simulink model "gm_sampleModel2013_4_sub"  (R2023a)
settings: Solver=VariableStepAuto  StartTime=0.0  StopTime=10.0  RelTol=1e-3
libraries: simulink x1
settings Model: Creator=user1  LastModifiedBy=user1
settings OptimizationCC: BlockReduction=off  ConditionallyExecuteInputs=off
settings DebuggingCC: InheritedTsInSrcMsg=none

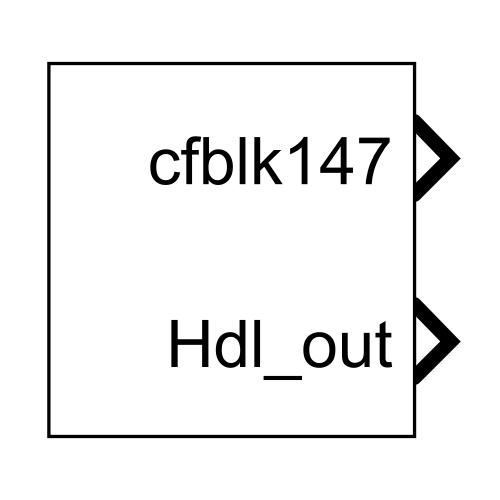
[thumbnail: Simulink's stored preview of the top-level diagram]
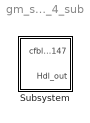
== system gm_sampleModel2013_4_sub ==
  Subsystem : Subsystem

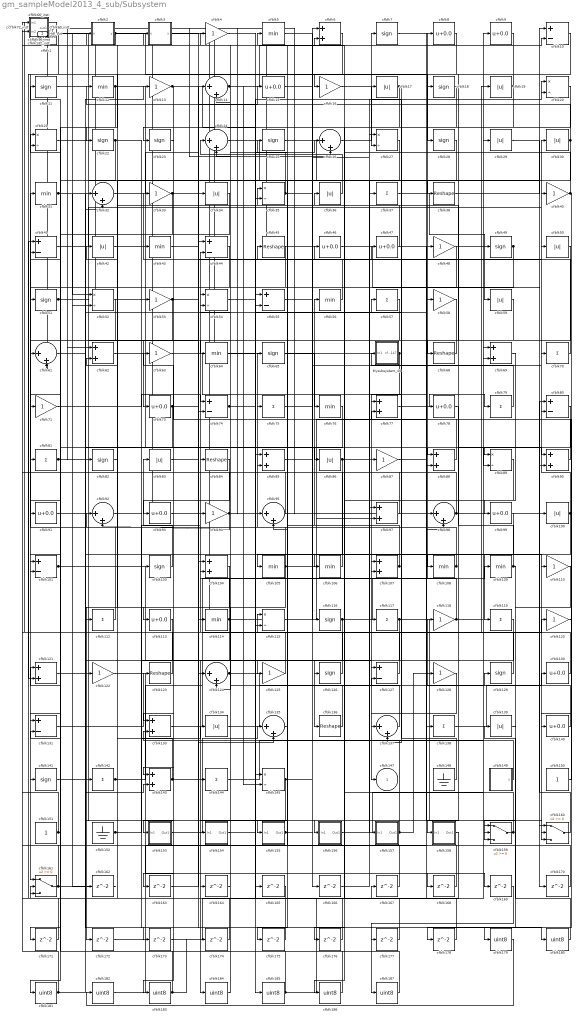
== system gm_sampleModel2013_4_sub/Subsystem ==
  Mysubsystem_45 : Subsystem
  cfblk1 : simulink/Logic and Bit Operations/Detect Increase  vinit=0.0  OutDataTypeStr=uint8
      settings: LibrarySourceBlock=|
      | hdlsllib/Logic and Bit
      | Operations/Detect
      | Increase
  cfblk{10,41,44,55,74,80,101,127,131} (9 alike) : Sum  Inputs=+-  OutDataTypeStr=uint8
  cfblk{17,19,29..30,34,36,42,50,59,83,86,100,134,139} (14 alike) : Abs  OutDataTypeStr=uint8  SaturateOnIntegerOverflow=off
  cfblk102_inst : Subsystem
  cfblk{7,11,18,22..23,25,28,49,51,65,82,103,116,126,129,141} (16 alike) : Signum
  cfblk{6,62,69,77,85,88,90,97,104,107,121,133,143} (13 alike) : Sum  OutDataTypeStr=uint8
  cfblk{5,12,31,43,56,64,76,105..106,108..109,114} (12 alike) : MinMax  OutDataTypeStr=uint8
  cfblk{4,13,16,33,40,48,53,58,63,71,87,94,110,118,120,122,125,128} (18 alike) : Gain  OutDataTypeStr=uint8
  cfblk111_inst : Subsystem
  cfblk{37,57,70,75,79,81,112,117,119,138,142,144} (12 alike) : Sum  Inputs=+  OutDataTypeStr=uint8
  cfblk{8..9,15,46..47,73,78,91,93,99,113,130,140} (13 alike) : Bias  Bias=0.0  SaturateOnIntegerOverflow=off
  cfblk{20..21,27,35,52,54,89,115,145} (9 alike) : Product  Inputs=*/  OutDataTypeStr=uint8  RndMeth=Zero  SaturateOnIntegerOverflow=on
  cfblk{38,45,68,84,123,136} (6 alike) : Reshape
  cfblk{14,24,26,32,61,92,95,98,124,135,137} (11 alike) : Sum  Inputs=|++  OutDataTypeStr=uint8
  cfblk132_inst : Subsystem
  cfblk148 : Ground
  cfblk149 : Subsystem  mask(Counter Limited){uplimit=double(7), tsamp=double(-1)}
      mask prompts: uplimit "Simulink:masks:UpperLimit_MP"; tsamp "Simulink:masks:SampleTime_MP"
      mask help: Simulink:masks:CounterLimited_MD
      mask init:
      | nbits = double(8);
      | tsamp = double(-1);
      | uplimit = double(7);
  cfblk150 : Constant  OutDataTypeStr=uint8  SampleTime=-1
  cfblk151 : Constant  OutDataTypeStr=uint8  SampleTime=-1
  cfblk152 : Ground
  cfblk153 : Subsystem
  cfblk154 : Subsystem
  cfblk155 : Subsystem
  cfblk156 : Subsystem
  cfblk157 : Subsystem
  cfblk158 : Subsystem
  cfblk159 : Switch  OutDataTypeStr=uint8  SaturateOnIntegerOverflow=off  InputSameDT=off
  cfblk160 : Switch  OutDataTypeStr=uint8  SaturateOnIntegerOverflow=off  InputSameDT=off
  cfblk161 : Switch  OutDataTypeStr=uint8  SaturateOnIntegerOverflow=off  InputSameDT=off
  cfblk{162..178} (17 alike) : Delay  SampleTime=1
  cfblk{179..187} (9 alike) : DataTypeConversion  OutDataTypeStr=uint8  SaturateOnIntegerOverflow=off  RndMeth=Floor
  cfblk2 : Subsystem  mask(Compare To Constant){relop=<=, const=double(3), OutDataTypeStr=uint8, ZeroCross=on}
      mask prompts: relop "Simulink:masks:Operator_MP"; const "Simulink:masks:ConstantValue_MP"; OutDataTypeStr "Simulink:masks:OutputDataType_MP"; ZeroCross "Simulink:masks:EnableZerocrossingDetection_MP"
      mask help: Simulink:masks:CompareToConstant_MD
      mask init:
      | OutDataTypeStr = 'uint8';
      | ZeroCross = 'on';
      | blkName = 'sampleModel2013_4_sub/Subsystem/cfblk2';
      | const = double(3);
      | const_str = '3.0';
      | const_val = double(3);
      | relop = '<=';
      | setValue = 'fixdt(0, 8)';
      | str = '<= 3';
      mask TypeOptions relop: == | ~= | < | <= | >= | >
      mask TypeOptions OutDataTypeStr: Simulink:masks:uint8 | Simulink:masks:boolean
      mask Callback ZeroCross: sl('zeroCrossEnable', gcbh);
      mask Display: disp(str)
  cfblk3 : Subsystem  mask(Compare To Constant){relop=<=, const=double(3), OutDataTypeStr=uint8, ZeroCross=on}
      mask prompts: relop "Simulink:masks:Operator_MP"; const "Simulink:masks:ConstantValue_MP"; OutDataTypeStr "Simulink:masks:OutputDataType_MP"; ZeroCross "Simulink:masks:EnableZerocrossingDetection_MP"
      mask help: Simulink:masks:CompareToConstant_MD
      mask init:
      | OutDataTypeStr = 'uint8';
      | ZeroCross = 'on';
      | blkName = 'sampleModel2013_4_sub/Subsystem/cfblk3';
      | const = double(3);
      | const_str = '3.0';
      | const_val = double(3);
      | relop = '<=';
      | setValue = 'fixdt(0, 8)';
      | str = '<= 3';
      mask TypeOptions relop: == | ~= | < | <= | >= | >
      mask TypeOptions OutDataTypeStr: Simulink:masks:uint8 | Simulink:masks:boolean
      mask Callback ZeroCross: sl('zeroCrossEnable', gcbh);
      mask Display: disp(str)
  cfblk39_inst : Subsystem
  cfblk60_inst : Subsystem
  cfblk66_inst : Subsystem
  cfblk72_inst : Subsystem
  cfblk96_inst : Subsystem
  cfblk147 : Outport  OutDataTypeStr=uint8  SampleTime=1  VectorParamsAs1DForOutWhenUnconnected=off
  Hdl_out : Outport  Port=2  OutDataTypeStr=uint8  SampleTime=1
  wires:
  Mysubsystem_45/1(cfblk147) -> Hdl_out/1, cfblk147/1
  cfblk1/1 -> cfblk161/1, cfblk159/3
  cfblk10/1 -> cfblk141/1
  cfblk100/1 -> cfblk30/1, cfblk160/3, cfblk119/1
  cfblk101/1 -> cfblk32/1, cfblk127/1
  cfblk102_inst/1(out1) -> cfblk82/1
  cfblk103/1 -> cfblk83/1
  cfblk104/1 -> cfblk172/1
  cfblk105/1 -> cfblk77/2, cfblk65/1, cfblk124/2
  cfblk106/1 -> cfblk75/1
  cfblk107/1 -> cfblk4/1, cfblk56/1
  cfblk108/1 -> cfblk85/2, cfblk2/1(u)
  cfblk109/1 -> cfblk19/1, cfblk35/1
  cfblk11/1 -> cfblk170/1
  cfblk110/1 -> cfblk159/2
  cfblk111_inst/1(out1) -> cfblk62/1
  cfblk112/1 -> cfblk31/1
  cfblk113/1 -> cfblk162/1
  cfblk114/1 -> cfblk44/2, cfblk142/1
  cfblk115/1 -> cfblk97/2
  cfblk116/1 -> cfblk136/1, cfblk109/1
  cfblk117/1 -> cfblk160/2, cfblk122/1
  cfblk118/1 -> cfblk29/1, cfblk24/1
  cfblk119/1 -> cfblk184/1
  cfblk12/1 -> cfblk91/1, cfblk89/1
  cfblk120/1 -> cfblk178/1
  cfblk121/1 -> cfblk13/1
  cfblk122/1 -> cfblk168/1
  cfblk123/1 -> cfblk21/1
  cfblk124/1 -> cfblk55/2, cfblk127/2
  cfblk125/1 -> cfblk115/1
  cfblk126/1 -> cfblk41/2
  cfblk127/1 -> cfblk96_inst/1(in1)
  cfblk128/1 -> cfblk137/1
  cfblk129/1 -> cfblk104/2
  cfblk13/1 -> cfblk165/1, cfblk153/1(In1)
  cfblk130/1 -> cfblk60_inst/1(in1)
  cfblk131/1 -> cfblk123/1
  cfblk132_inst/1(out1) -> cfblk95/1, cfblk39_inst/2(in2)
  cfblk133/1 -> cfblk8/1
  cfblk134/1 -> cfblk129/1
  cfblk135/1 -> cfblk5/1
  cfblk136/1 -> cfblk24/2
  cfblk137/1 -> cfblk60_inst/2(in2)
  cfblk138/1 -> cfblk130/1
  cfblk139/1 -> cfblk179/1
  cfblk14/1 -> cfblk10/2, cfblk145/2
  cfblk140/1 -> cfblk118/1
  cfblk141/1 -> cfblk156/1(In1)
  cfblk142/1 -> cfblk120/1, cfblk37/1
  cfblk143/1 -> cfblk92/1, cfblk135/1
  cfblk144/1 -> cfblk69/1
  cfblk145/1 -> cfblk6/1, cfblk164/1
  cfblk148/1 -> cfblk55/1
  cfblk149/1(y) -> cfblk133/2
  cfblk15/1 -> cfblk116/1
  cfblk150/1 -> cfblk80/2
  cfblk151/1 -> cfblk132_inst/2(in2), cfblk121/1
  cfblk152/1 -> cfblk134/1, cfblk94/1
  cfblk153/1(Out1) -> cfblk20/1
  cfblk154/1(Out1) -> cfblk85/1
  cfblk155/1(Out1) -> cfblk166/1, cfblk70/1
  cfblk156/1(Out1) -> cfblk9/1
  cfblk157/1(Out1) -> cfblk104/1, cfblk128/1
  cfblk158/1(Out1) -> cfblk167/1
  cfblk159/1 -> cfblk97/1, cfblk36/1
  cfblk16/1 -> cfblk27/2
  cfblk160/1 -> cfblk80/1
  cfblk161/1 -> cfblk72_inst/1(in1), cfblk143/2
  cfblk162/1 -> cfblk1/1
  cfblk163/1 -> cfblk124/1
  cfblk164/1 -> cfblk14/2
  cfblk165/1 -> cfblk161/2
  cfblk166/1 -> cfblk20/2
  cfblk167/1 -> cfblk72_inst/2(in2)
  cfblk168/1 -> cfblk102_inst/1(in1)
  cfblk169/1 -> cfblk187/1
  cfblk17/1 -> cfblk137/2, cfblk35/2
  cfblk170/1 -> cfblk95/2
  cfblk171/1 -> cfblk161/3
  cfblk172/1 -> cfblk88/2
  cfblk173/1 -> cfblk69/2
  cfblk174/1 -> cfblk66_inst/1(in1)
  cfblk175/1 -> cfblk41/1
  cfblk176/1 -> cfblk145/1
  cfblk177/1 -> cfblk6/2
  cfblk178/1 -> cfblk62/2
  cfblk179/1 -> cfblk182/1
  cfblk18/1 -> cfblk106/1
  cfblk180/1 -> cfblk139/1
  cfblk181/1 -> cfblk132_inst/1(in1), cfblk57/1
  cfblk182/1 -> cfblk34/1
  cfblk183/1 -> cfblk21/2, cfblk174/1
  cfblk184/1 -> cfblk84/1
  cfblk185/1 -> cfblk131/2, cfblk48/1
  cfblk186/1 -> cfblk54/1
  cfblk187/1 -> cfblk54/2
  cfblk19/1 -> cfblk77/1, cfblk16/1
  cfblk2/1(y) -> cfblk66_inst/2(in2), cfblk28/1
  cfblk20/1 -> cfblk23/1
  cfblk21/1 -> cfblk103/1
  cfblk22/1 -> cfblk61/1, cfblk126/1, cfblk177/1
  cfblk23/1 -> cfblk143/1
  cfblk24/1 -> cfblk87/1
  cfblk25/1 -> cfblk157/1(In1)
  cfblk26/1 -> cfblk7/1
  cfblk27/1 -> cfblk155/1(In1)
  cfblk28/1 -> cfblk112/1
  cfblk29/1 -> cfblk160/1
  cfblk3/1(y) -> cfblk180/1
  cfblk30/1 -> cfblk175/1, cfblk12/1
  cfblk31/1 -> cfblk131/1, cfblk52/1, cfblk173/1
  cfblk32/1 -> cfblk15/1
  cfblk33/1 -> cfblk14/1, cfblk101/2
  cfblk34/1 -> cfblk181/1
  cfblk35/1 -> cfblk111_inst/1(in1), cfblk89/2
  cfblk36/1 -> cfblk96_inst/2(in2)
  cfblk37/1 -> cfblk59/1
  cfblk38/1 -> cfblk10/1
  cfblk39_inst/1(out1) -> cfblk61/2, cfblk49/1
  cfblk4/1 -> cfblk88/1
  cfblk40/1 -> cfblk140/1, cfblk3/1(u)
  cfblk41/1 -> cfblk40/1
  cfblk42/1 -> cfblk33/1
  cfblk43/1 -> cfblk74/2
  cfblk44/1 -> cfblk163/1
  cfblk45/1 -> cfblk51/1
  cfblk46/1 -> cfblk90/2
  cfblk47/1 -> cfblk102_inst/2(in2)
  cfblk48/1 -> cfblk115/2
  cfblk49/1 -> cfblk186/1, cfblk107/2
  cfblk5/1 -> cfblk38/1
  cfblk50/1 -> cfblk133/1
  cfblk51/1 -> cfblk32/2, cfblk144/1
  cfblk52/1 -> cfblk171/1
  cfblk53/1 -> cfblk73/1, cfblk135/2
  cfblk54/1 -> cfblk185/1
  cfblk55/1 -> cfblk18/1
  cfblk56/1 -> cfblk43/1
  cfblk57/1 -> cfblk71/1
  cfblk58/1 -> cfblk93/1
  cfblk59/1 -> cfblk107/1
  cfblk6/1 -> cfblk22/1
  cfblk60_inst/1(out1) -> cfblk117/1
  cfblk61/1 -> cfblk86/1
  cfblk62/1 -> cfblk114/1
  cfblk63/1 -> cfblk98/2
  cfblk64/1 -> cfblk90/1
  cfblk65/1 -> cfblk76/1
  cfblk66_inst/1(out1) -> cfblk26/2, cfblk100/1
  cfblk68/1 -> cfblk64/1
  cfblk69/1 -> cfblk99/1
  cfblk7/1 -> cfblk138/1
  cfblk70/1 -> cfblk46/1
  cfblk71/1 -> cfblk74/1
  cfblk72_inst/1(out1) -> cfblk53/1
  cfblk73/1 -> cfblk45/1, cfblk101/1
  cfblk74/1 -> cfblk50/1, cfblk26/1
  cfblk75/1 -> cfblk58/1
  cfblk76/1 -> cfblk113/1
  cfblk77/1 -> cfblk79/1
  cfblk78/1 -> cfblk108/1
  cfblk79/1 -> cfblk17/1
  cfblk8/1 -> cfblk121/2
  cfblk80/1 -> cfblk158/1(In1)
  cfblk81/1 -> cfblk11/1, cfblk52/2
  cfblk82/1 -> cfblk42/1
  cfblk83/1 -> cfblk169/1
  cfblk84/1 -> cfblk183/1
  cfblk85/1 -> cfblk27/1
  cfblk86/1 -> cfblk78/1, cfblk125/1
  cfblk87/1 -> cfblk159/1
  cfblk88/1 -> cfblk25/1
  cfblk89/1 -> cfblk176/1
  cfblk9/1 -> cfblk68/1
  cfblk90/1 -> cfblk63/1
  cfblk91/1 -> cfblk110/1
  cfblk92/1 -> cfblk154/1(In1)
  cfblk93/1 -> cfblk47/1
  cfblk94/1 -> cfblk92/2, cfblk111_inst/2(in2)
  cfblk95/1 -> cfblk39_inst/1(in1)
  cfblk96_inst/1(out1) -> cfblk98/1
  cfblk97/1 -> cfblk81/1
  cfblk98/1 -> cfblk44/1, Mysubsystem_45/1(In1)
  cfblk99/1 -> cfblk105/1

== system gm_sampleModel2013_4_sub/Subsystem/Mysubsystem_45 ==
  In1 : Inport  OutDataTypeStr=uint8  PortDimensions=1  SampleTime=1
  cfblk67 : MinMax
  cfblk147 : Outport  SampleTime=1  VectorParamsAs1DForOutWhenUnconnected=off
  wires:
  In1/1 -> cfblk67/1
  cfblk67/1 -> cfblk147/1

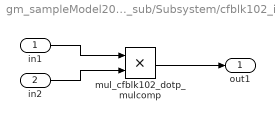
== system gm_sampleModel2013_4_sub/Subsystem/cfblk102_inst ==
  in1 : Inport  OutDataTypeStr=uint8  SampleTime=1
  in2 : Inport  Port=2  OutDataTypeStr=uint8  SampleTime=1
  mul_cfblk102_dotp_mulcomp : Product  Inputs=**  OutDataTypeStr=uint8  SampleTime=1
  out1 : Outport  OutDataTypeStr=uint8  SampleTime=1
  wires:
  in1/1 -> mul_cfblk102_dotp_mulcomp/1
  in2/1 -> mul_cfblk102_dotp_mulcomp/2
  mul_cfblk102_dotp_mulcomp/1 -> out1/1

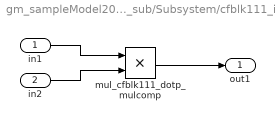
== system gm_sampleModel2013_4_sub/Subsystem/cfblk111_inst ==
  in1 : Inport  OutDataTypeStr=uint8  SampleTime=1
  in2 : Inport  Port=2  OutDataTypeStr=uint8  SampleTime=1
  mul_cfblk111_dotp_mulcomp : Product  Inputs=**  OutDataTypeStr=uint8  SampleTime=1
  out1 : Outport  OutDataTypeStr=uint8  SampleTime=1
  wires:
  in1/1 -> mul_cfblk111_dotp_mulcomp/1
  in2/1 -> mul_cfblk111_dotp_mulcomp/2
  mul_cfblk111_dotp_mulcomp/1 -> out1/1

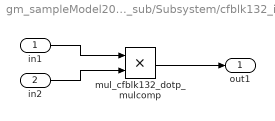
== system gm_sampleModel2013_4_sub/Subsystem/cfblk132_inst ==
  in1 : Inport  OutDataTypeStr=uint8  SampleTime=1
  in2 : Inport  Port=2  OutDataTypeStr=uint8  SampleTime=1
  mul_cfblk132_dotp_mulcomp : Product  Inputs=**  OutDataTypeStr=uint8  SampleTime=1
  out1 : Outport  OutDataTypeStr=uint8  SampleTime=1
  wires:
  in1/1 -> mul_cfblk132_dotp_mulcomp/1
  in2/1 -> mul_cfblk132_dotp_mulcomp/2
  mul_cfblk132_dotp_mulcomp/1 -> out1/1

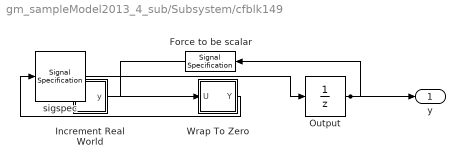
== system gm_sampleModel2013_4_sub/Subsystem/cfblk149 ==
  Force to be scalar : SignalSpecification  DisableCoverage=on  Dimensions=1
  Increment Real World : Subsystem  mask(Real World Value Increment){}
      mask help: Simulink:masks:RealWorldValueIncrement_MD
      mask Display: disp('V++')
  Output : UnitDelay  InitialCondition=0.0  SampleTime=tsamp  HasFrameUpgradeWarning=on
  Wrap To Zero : Subsystem  mask(Wrap To Zero){Threshold=double(7)}
      mask prompts: Threshold "Simulink:masks:Threshold_MP"
      mask help: Simulink:masks:WrapToZero_MD
  sigspec : SignalSpecification  OutDataTypeStr=uint8  Dimensions=1
  y : Outport  SampleTime=1
  wires:
  Force to be scalar/1 -> Increment Real World/1(u)
  Increment Real World/1(y) -> Wrap To Zero/1(U)
  Output/1 -> Force to be scalar/1, y/1
  Wrap To Zero/1(Y) -> sigspec/1
  sigspec/1 -> Output/1

== system gm_sampleModel2013_4_sub/Subsystem/cfblk153 ==
  In1 : Inport  OutDataTypeStr=uint8  PortDimensions=1  SampleTime=1
  Out1 : Outport  SampleTime=1
  wires:
  In1/1 -> Out1/1

== system gm_sampleModel2013_4_sub/Subsystem/cfblk154 ==
  In1 : Inport  OutDataTypeStr=uint8  PortDimensions=1  SampleTime=1
  Out1 : Outport  SampleTime=1
  wires:
  In1/1 -> Out1/1

== system gm_sampleModel2013_4_sub/Subsystem/cfblk155 ==
  In1 : Inport  OutDataTypeStr=uint8  PortDimensions=1  SampleTime=1
  Out1 : Outport  SampleTime=1
  wires:
  In1/1 -> Out1/1

== system gm_sampleModel2013_4_sub/Subsystem/cfblk156 ==
  In1 : Inport  OutDataTypeStr=uint8  PortDimensions=1  SampleTime=1
  Out1 : Outport  SampleTime=1
  wires:
  In1/1 -> Out1/1

== system gm_sampleModel2013_4_sub/Subsystem/cfblk157 ==
  In1 : Inport  OutDataTypeStr=uint8  PortDimensions=1  SampleTime=1
  Out1 : Outport  SampleTime=1
  wires:
  In1/1 -> Out1/1

== system gm_sampleModel2013_4_sub/Subsystem/cfblk158 ==
  In1 : Inport  OutDataTypeStr=uint8  PortDimensions=1  SampleTime=1
  Out1 : Outport  SampleTime=1
  wires:
  In1/1 -> Out1/1

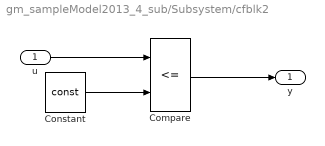
== system gm_sampleModel2013_4_sub/Subsystem/cfblk2 ==
  u : Inport  OutDataTypeStr=uint8  SampleTime=1
  Compare : RelationalOperator  Operator=<=  OutDataTypeStr=fixdt(0, 8)
  Constant : Constant  DisableCoverage=on  Value=const  OutDataTypeStr=Inherit: Inherit via back propagation  SampleTime=-1
  y : Outport  SampleTime=1
  wires:
  u/1 -> Compare/1
  Compare/1 -> y/1
  Constant/1 -> Compare/2

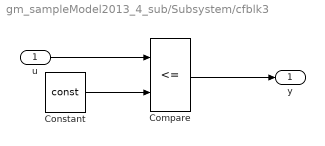
== system gm_sampleModel2013_4_sub/Subsystem/cfblk3 ==
  u : Inport  OutDataTypeStr=uint8  SampleTime=1
  Compare : RelationalOperator  Operator=<=  OutDataTypeStr=fixdt(0, 8)
  Constant : Constant  DisableCoverage=on  Value=const  OutDataTypeStr=Inherit: Inherit via back propagation  SampleTime=-1
  y : Outport  SampleTime=1
  wires:
  u/1 -> Compare/1
  Compare/1 -> y/1
  Constant/1 -> Compare/2

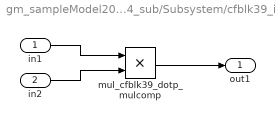
== system gm_sampleModel2013_4_sub/Subsystem/cfblk39_inst ==
  in1 : Inport  OutDataTypeStr=uint8  SampleTime=1
  in2 : Inport  Port=2  OutDataTypeStr=uint8  SampleTime=1
  mul_cfblk39_dotp_mulcomp : Product  Inputs=**  OutDataTypeStr=uint8  SampleTime=1
  out1 : Outport  OutDataTypeStr=uint8  SampleTime=1
  wires:
  in1/1 -> mul_cfblk39_dotp_mulcomp/1
  in2/1 -> mul_cfblk39_dotp_mulcomp/2
  mul_cfblk39_dotp_mulcomp/1 -> out1/1

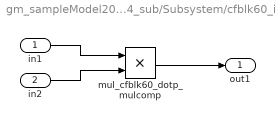
== system gm_sampleModel2013_4_sub/Subsystem/cfblk60_inst ==
  in1 : Inport  OutDataTypeStr=uint8  SampleTime=1
  in2 : Inport  Port=2  OutDataTypeStr=uint8  SampleTime=1
  mul_cfblk60_dotp_mulcomp : Product  Inputs=**  OutDataTypeStr=uint8  SampleTime=1
  out1 : Outport  OutDataTypeStr=uint8  SampleTime=1
  wires:
  in1/1 -> mul_cfblk60_dotp_mulcomp/1
  in2/1 -> mul_cfblk60_dotp_mulcomp/2
  mul_cfblk60_dotp_mulcomp/1 -> out1/1

== system gm_sampleModel2013_4_sub/Subsystem/cfblk66_inst ==
  in1 : Inport  OutDataTypeStr=uint8  SampleTime=1
  in2 : Inport  Port=2  OutDataTypeStr=uint8  SampleTime=1
  mul_cfblk66_dotp_mulcomp : Product  Inputs=**  OutDataTypeStr=uint8  SampleTime=1
  out1 : Outport  OutDataTypeStr=uint8  SampleTime=1
  wires:
  in1/1 -> mul_cfblk66_dotp_mulcomp/1
  in2/1 -> mul_cfblk66_dotp_mulcomp/2
  mul_cfblk66_dotp_mulcomp/1 -> out1/1

== system gm_sampleModel2013_4_sub/Subsystem/cfblk72_inst ==
  in1 : Inport  OutDataTypeStr=uint8  SampleTime=1
  in2 : Inport  Port=2  OutDataTypeStr=uint8  SampleTime=1
  mul_cfblk72_dotp_mulcomp : Product  Inputs=**  OutDataTypeStr=uint8  SampleTime=1
  out1 : Outport  OutDataTypeStr=uint8  SampleTime=1
  wires:
  in1/1 -> mul_cfblk72_dotp_mulcomp/1
  in2/1 -> mul_cfblk72_dotp_mulcomp/2
  mul_cfblk72_dotp_mulcomp/1 -> out1/1

== system gm_sampleModel2013_4_sub/Subsystem/cfblk96_inst ==
  in1 : Inport  OutDataTypeStr=uint8  SampleTime=1
  in2 : Inport  Port=2  OutDataTypeStr=uint8  SampleTime=1
  mul_cfblk96_dotp_mulcomp : Product  Inputs=**  OutDataTypeStr=uint8  SampleTime=1
  out1 : Outport  OutDataTypeStr=uint8  SampleTime=1
  wires:
  in1/1 -> mul_cfblk96_dotp_mulcomp/1
  in2/1 -> mul_cfblk96_dotp_mulcomp/2
  mul_cfblk96_dotp_mulcomp/1 -> out1/1

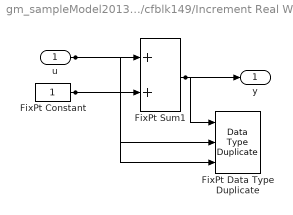
== system gm_sampleModel2013_4_sub/Subsystem/cfblk149/Increment Real World ==
  u : Inport  OutDataTypeStr=uint8  SampleTime=1
  FixPt Constant : Constant  DisableCoverage=on  OutDataTypeStr=Inherit: Inherit via back propagation  SampleTime=-1
  FixPt Data Type Duplicate : DataTypeDuplicate  DisableCoverage=on  NumInputPorts=3
  FixPt Sum1 : Sum  InputSameDT=on  OutDataTypeStr=Inherit: Inherit via back propagation  LockScale=on
  y : Outport  SampleTime=1
  wires:
  u/1 -> FixPt Sum1/1, FixPt Data Type Duplicate/2
  FixPt Constant/1 -> FixPt Sum1/2, FixPt Data Type Duplicate/3
  FixPt Sum1/1 -> FixPt Data Type Duplicate/1, y/1

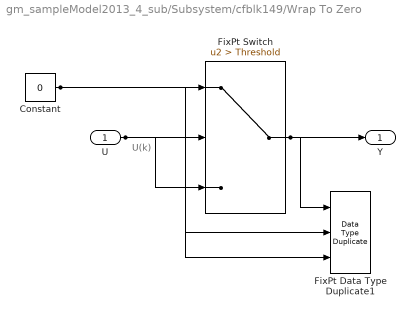
== system gm_sampleModel2013_4_sub/Subsystem/cfblk149/Wrap To Zero ==
  note: U(k)
  U : Inport  OutDataTypeStr=uint8  SampleTime=1
  Constant : Constant  DisableCoverage=on  Value=0  OutDataTypeStr=Inherit: Inherit via back propagation  SampleTime=-1
  FixPt Data Type Duplicate1 : DataTypeDuplicate  DisableCoverage=on  NumInputPorts=3
  FixPt Switch : Switch  Criteria=u2 > Threshold  Threshold=Threshold  OutDataTypeStr=Inherit: Inherit via back propagation  ZeroCross=off  SaturateOnIntegerOverflow=off  InputSameDT=off
  Y : Outport  SampleTime=1
  wires:
  U/1 -> FixPt Switch/3, FixPt Switch/2, FixPt Data Type Duplicate1/2
  Constant/1 -> FixPt Switch/1, FixPt Data Type Duplicate1/3
  FixPt Switch/1 -> FixPt Data Type Duplicate1/1, Y/1
